simulink model "Copy_of_LTI"  (Simulink 7.8)
settings: Solver=ode45  StartTime=0.0  StopTime=10.0  RelTol=1e-3
undefined symbols (not defined in the file): A, B, C, D, var, x0
settings Model: Creator=chepeadan  LastModifiedBy=Tigervilla
settings DebuggingCC: FcnCallInpInsideContextMsg=Use local settings  StrictBusMsg=Warning

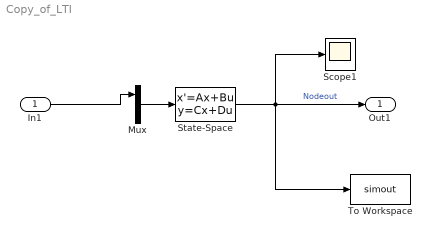
== system Copy_of_LTI ==
  In1 : Inport
  Mux : Mux  Inputs=2
  Scope1 : Scope
      settings: TimeRange=0.5847953216374258  YMin=-0.1657458563535892  YMax=1.21546961325967
  State-Space : StateSpace  A=A  B=B  C=C  D=D  X0=x0+var*rand(1)
  To Workspace : ToWorkspace  VariableName=simout  SampleTime=-1  SaveFormat=Structure With Time
  Out1 : Outport
  wires:
  Mux/1 -> State-Space/1
  In1/1 -> Mux/1
  State-Space/1 -> Out1/1, Scope1/1, To Workspace/1  "Nodeout"
